simulink model "AN_Simulink_Model_v1"  (R2019b)
settings: Solver=VariableStepAuto  StartTime=0.0  StopTime=testtime  RelTol=1e-3
InitFcn:
  | AN_InitFcn_Callback
StopFcn:
  | AN_StopFcn_Callback
values from neighbouring files (symbols this model uses):
  alpha1 = 1.5e-6*100e3    (= 0.15)    [AN_Get_Model_Parameters.m]
  alpha2 = 1e-2*100e3    (= 1000)    [AN_Get_Model_Parameters.m]
  C1initphase = C1initphase + atan(CF/(-rzero))-atan((CF-pimag(2*i-1))/(-preal(2*i-1)))-atan((CF+pimag(2*i-1))/(-preal(2*i-1)))    [AN_Get_Model_Parameters.m]
  c1LPihc = ( Cihc - 2*pi*Fcihc ) / ( Cihc + 2*pi*Fcihc )    [AN_Get_Model_Parameters.m]
  c1LPohc = ( Cohc - 2*pi*Fcohc ) / ( Cohc + 2*pi*Fcohc )    [AN_Get_Model_Parameters.m]
  C1slope = 0.1    [AN_Get_Model_Parameters.m]
  c2LPihc = 2*pi*Fcihc / (2*pi*Fcihc + Cihc)    [AN_Get_Model_Parameters.m]
  c2LPohc = 2*pi*Fcohc / (2*pi*Fcohc + Cohc)    [AN_Get_Model_Parameters.m]
  C2slope = 0.2    [AN_Get_Model_Parameters.m]
  centerfreq = 165.4*(10^((bmplace+1.2)/(35/2.1)) - 1.0)    [AN_Get_Model_Parameters.m]
  CF = 2*pi*cf    [AN_Get_Model_Parameters.m]
  cf_factor = min(cfsat, 10^(cfslope*cf/1e3 + cfconst)) * 2.0    [AN_Get_Model_Parameters.m]
  cordiciterationswb = 52    [AN_Get_Model_Parameters.m]
  delta_phase = -2*pi*centerfreq*tdres    [AN_Get_Model_Parameters.m]
  fs_bilinear = 2*pi*cf/tan(2*pi*cf*tdres/2)    [AN_Get_Model_Parameters.m]
  gainihc = 1.0    (= 1)    [AN_Get_Model_Parameters.m]
  gainohc = 1.0    (= 1)    [AN_Get_Model_Parameters.m]
  ihcasym = 3.0    (= 3)    [AN_Get_Model_Parameters.m]
  m11 = 1/(C^2+5.9761e+003*C+2.5255e+007)    [AN_Get_Model_Parameters.m]
  m12 = -2*C^2+2*2.5255e+007    [AN_Get_Model_Parameters.m]
  m13 = C^2-5.9761e+003*C+2.5255e+007    [AN_Get_Model_Parameters.m]
  m14 = C^2+5.6665e+003*C    [AN_Get_Model_Parameters.m]
  m15 = -2*C^2    [AN_Get_Model_Parameters.m]
  m16 = C^2-5.6665e+003*C    [AN_Get_Model_Parameters.m]
  m21 = 1/(C^2+6.4255e+003*C+1.3975e+008)    [AN_Get_Model_Parameters.m]
  m22 = -2*C^2+2*1.3975e+008    [AN_Get_Model_Parameters.m]
  m23 = C^2-6.4255e+003*C+1.3975e+008    [AN_Get_Model_Parameters.m]
  m24 = C^2+5.8934e+003*C+1.7926e+008    [AN_Get_Model_Parameters.m]
  m25 = -2*C^2+2*1.7926e+008    [AN_Get_Model_Parameters.m]
  m26 = C^2-5.8934e+003*C+1.7926e+008    [AN_Get_Model_Parameters.m]
  m31 = 1/(C^2+2.4891e+004*C+1.2700e+009)    [AN_Get_Model_Parameters.m]
  m32 = -2*C^2+2*1.2700e+009    [AN_Get_Model_Parameters.m]
  m33 = C^2-2.4891e+004*C+1.2700e+009    [AN_Get_Model_Parameters.m]
  m34 = (3.1137e+003*C+6.9768e+008)    [AN_Get_Model_Parameters.m]
  m35 = 2*6.9768e+008    (= 1395360000)    [AN_Get_Model_Parameters.m]
  m36 = -3.1137e+003*C+6.9768e+008    [AN_Get_Model_Parameters.m]
  megainmax = 2    [AN_Get_Model_Parameters.m]
  minR = 0.05    [AN_Get_Model_Parameters.m]
  multFac = max(2.95*max(1.0,1.5-spont/100), 4.3-0.2*cf/1e3)    [AN_Get_Model_Parameters.m]
  norm_gainc1 = single(norm_gainc1)    [AN_Get_Model_Parameters.m]
  nSites = single(4)    [AN_Get_Model_Parameters.m]
  ohcasym = 7.0    (= 7)    [AN_Get_Model_Parameters.m]
  order_of_zero = half_order_pole    (= 5)    [AN_Get_Model_Parameters.m]
  pimag = zeros(11,1)    [AN_Get_Model_Parameters.m]
  preal = zeros(11,1)    [AN_Get_Model_Parameters.m]
  s0 = 12.0    (= 12)    [AN_Get_Model_Parameters.m]
  s1 = 5.0    (= 5)    [AN_Get_Model_Parameters.m]
  shift = 1.0/(1.0+ohcasym)    (= 0.125)    [AN_Get_Model_Parameters.m]
  spont = 100    [AN_Get_Model_Parameters.m]
  strength = (20.0e6)/(10^(corner/20))    (= 2000)    [AN_Get_Model_Parameters.m]
  tauwb = TauWBMax + (bmTaubm-bmTaumax)*(TauWBMax-TauWBMin)/(bmTaumax-bmTaumin)    [AN_Get_Model_Parameters.m]
  TauWBMax = Taumin + 0.2*(Taumax-Taumin)    [AN_Get_Model_Parameters.m]
  TauWBMin = TauWBMax/Taumax*Taumin    [AN_Get_Model_Parameters.m]
  wborder = 3    [AN_Get_Model_Parameters.m]
  x0 = s0*log((1.0/shift-1)/(1+exp(x1/s1)))    [AN_Get_Model_Parameters.m]
  x1 = 5.0    (= 5)    [AN_Get_Model_Parameters.m]
undefined symbols (not defined in the file or in its folder): bmTaumax, bmTaumin, cf, cihc, cohc, dfilt, Fs, jsin, norm_gainc2, tabs, tdres, trel, wbgain
libraries: dsparch4 x7, simulink x6, dspsrcs4 x3
(part 2 of 2)

== system AN_Simulink_Model_v1/Auditory Nerve Model/Subsystem/IHC LP Filter ==
  stimulus : Inport  OutDataTypeStr=single
  Biquad Filter1 : dsparch4/Biquad Filter  FilterSource=Dialog parameters  CoeffSource=Specify via dialog  FilterObject=dfilt.df2tsos([1 0.3 0.4],[1 0.1 0.2])  IIRFiltStruct=Direct form II transposed  BiQuadCoeffs=[c2LPihc c2LPihc 0 1 -c1LPihc 0; c2LPihc c2LPihc 0 1 -c1LPihc 0; c2LPihc c2LPihc 0 1 -c1LPihc 0]  ScaleValues=1  IC=0  ICnum=0  ICden=0  a0Flag=Warning  optimizeScaleValues=on  ScaleValueMode=Specify via input port (g)  roundingMode=Floor  overflowMode=on  scaleValueFracLength=14  denProdOutputFracLength=30  denAccumFracLength=30  secondMemoryFracLength=15
      settings: SourceProductName=DSP System Toolbox
  Biquad Filter4 : dsparch4/Biquad Filter  FilterSource=Dialog parameters  CoeffSource=Specify via dialog  FilterObject=dfilt.df2tsos([1 0.3 0.4],[1 0.1 0.2])  IIRFiltStruct=Direct form II transposed  BiQuadCoeffs=[gainihc*c2LPihc gainihc*c2LPihc 0 1 -c1LPihc 0; c2LPihc c2LPihc 0 1 -c1LPihc 0; c2LPihc c2LPihc 0 1 -c1LPihc 0;c2LPihc c2LPihc 0 1 -c1LPihc 0]  ScaleValues=1  IC=0  ICnum=0  ICden=0  a0Flag=Warning  optimizeScaleValues=on  ScaleValueMode=Specify via input port (g)  roundingMode=Floor  overflowMode=on  scaleValueFracLength=14  denProdOutputFracLength=30  denAccumFracLength=30  secondMemoryFracLength=15
      settings: SourceProductName=DSP System Toolbox
  output : Outport  VectorParamsAs1DForOutWhenUnconnected=off
  wires:
  stimulus/1 -> Biquad Filter4/1
  Biquad Filter4/1 -> Biquad Filter1/1  "output"
  Biquad Filter1/1 -> output/1  "output"

== system AN_Simulink_Model_v1/Auditory Nerve Model/Subsystem1/Calculate tauc1 ==
  note: Calculate final Time Constant which will be fed forward into C1 filter
  In1 : Inport
  Add : Sum
  Constant : Constant  Value=cohc  OutDataTypeStr=single  SampleTime=-1
  Constant1 : Constant  Value=bmTaumin  OutDataTypeStr=single  SampleTime=-1
  Constant2 : Constant  Value=bmTaumin  OutDataTypeStr=single  SampleTime=-1
  Product : Product
  Subtract : Sum  Inputs=+-
  Out1 : Outport  VectorParamsAs1DForOutWhenUnconnected=off
  wires:
  In1/1 -> Subtract/1  "tmptauc1"
  Constant/1 -> Product/1
  Constant1/1 -> Subtract/2
  Product/1 -> Add/1
  Add/1 -> Out1/1  "tauc1"
  Subtract/1 -> Product/2
  Constant2/1 -> Add/2

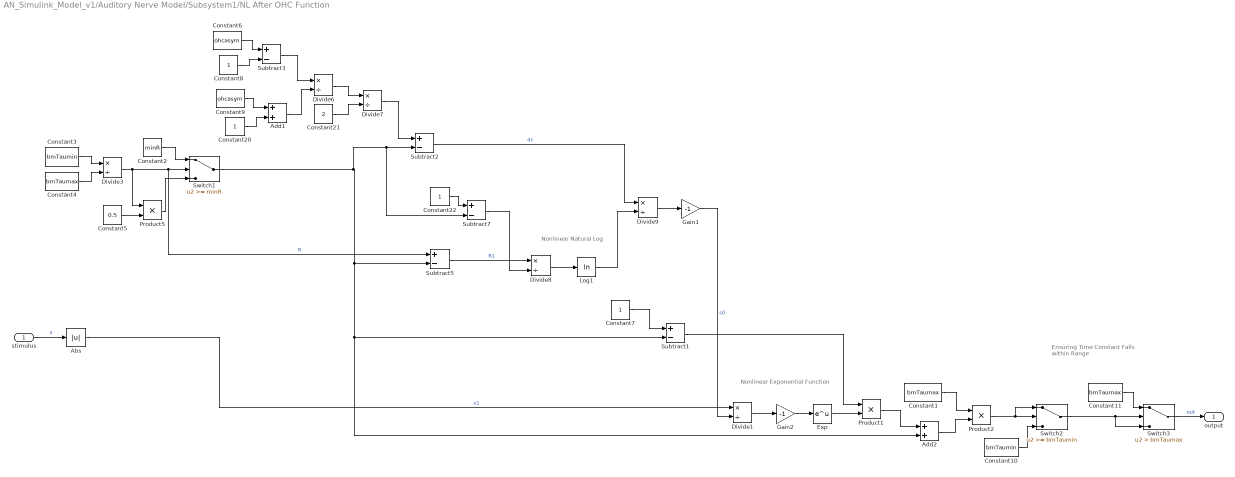
== system AN_Simulink_Model_v1/Auditory Nerve Model/Subsystem1/NL After OHC Function ==
  note: Ensuring Time Constant Falls within Range
  note: Nonlinear Natural Log
  note: Nonlinear Exponential Function
  stimulus : Inport
  Abs : Abs
  Add1 : Sum
  Add2 : Sum
  Constant1 : Constant  Value=bmTaumax  OutDataTypeStr=single  SampleTime=-1
  Constant10 : Constant  Value=bmTaumin  OutDataTypeStr=single  SampleTime=-1
  Constant11 : Constant  Value=bmTaumax  OutDataTypeStr=single  SampleTime=-1
  Constant2 : Constant  Value=minR  OutDataTypeStr=single  SampleTime=-1
  Constant{7..8,20,22} (4 alike) : Constant  OutDataTypeStr=single  SampleTime=-1
  Constant21 : Constant  Value=2  OutDataTypeStr=single  SampleTime=-1
  Constant3 : Constant  Value=bmTaumin  OutDataTypeStr=single  SampleTime=-1
  Constant4 : Constant  Value=bmTaumax  OutDataTypeStr=single  SampleTime=-1
  Constant5 : Constant  Value=0.5  OutDataTypeStr=single  SampleTime=-1
  Constant6 : Constant  Value=ohcasym  OutDataTypeStr=single  SampleTime=-1
  Constant9 : Constant  Value=ohcasym  OutDataTypeStr=single  SampleTime=-1
  Divide{1,3,6..9} (6 alike) : Product  Inputs=*/  SaturateOnIntegerOverflow=on  RndMeth=Zero
  Exp : Math  SaturateOnIntegerOverflow=on
  Gain1 : Gain  Gain=-1
  Gain2 : Gain  Gain=-1
  Log1 : Math  Operator=log  SaturateOnIntegerOverflow=on
  Product1 : Product
  Product2 : Product
  Product5 : Product
  Subtract{1..3,5,7} (5 alike) : Sum  Inputs=+-
  Switch1 : Switch  Threshold=minR
  Switch2 : Switch  Threshold=bmTaumin
  Switch3 : Switch  Criteria=u2 > Threshold  Threshold=bmTaumax
  output : Outport  VectorParamsAs1DForOutWhenUnconnected=off
  wires:
  Constant3/1 -> Divide3/1
  Constant4/1 -> Divide3/2
  Divide3/1 -> Subtract5/1, Switch1/2, Product5/1  "R"
  Constant2/1 -> Switch1/1
  Constant5/1 -> Product5/2
  Product5/1 -> Switch1/3
  Switch1/1 -> Subtract7/2, Subtract2/2, Add2/2, Subtract1/2, Subtract5/2
  Constant8/1 -> Subtract3/2
  Constant6/1 -> Subtract3/1
  Constant20/1 -> Add1/2
  Constant9/1 -> Add1/1
  Subtract3/1 -> Divide6/1
  Add1/1 -> Divide6/2
  Divide6/1 -> Divide7/1
  Constant21/1 -> Divide7/2
  Divide7/1 -> Subtract2/1
  Subtract2/1 -> Divide9/1  "dc"
  Subtract5/1 -> Divide8/1  "R1"
  Constant22/1 -> Subtract7/1
  Subtract7/1 -> Divide8/2
  Divide8/1 -> Log1/1
  Log1/1 -> Divide9/2
  Divide9/1 -> Gain1/1
  Gain1/1 -> Divide1/2  "s0"
  stimulus/1 -> Abs/1  "x"
  Abs/1 -> Divide1/1  "x1"
  Constant7/1 -> Subtract1/1
  Divide1/1 -> Gain2/1
  Gain2/1 -> Exp/1
  Subtract1/1 -> Product1/1
  Exp/1 -> Product1/2
  Product1/1 -> Add2/1
  Constant1/1 -> Product2/1
  Add2/1 -> Product2/2
  Product2/1 -> Switch2/1, Switch2/2
  Constant10/1 -> Switch2/3
  Switch2/1 -> Switch3/3, Switch3/2
  Constant11/1 -> Switch3/1
  Switch3/1 -> output/1  "out"

== system AN_Simulink_Model_v1/Auditory Nerve Model/Subsystem1/OHC LP Filter ==
  stimulus : Inport
  Biquad Filter4 : dsparch4/Biquad Filter  FilterSource=Dialog parameters  CoeffSource=Specify via dialog  FilterObject=dfilt.df2tsos([1 0.3 0.4],[1 0.1 0.2])  IIRFiltStruct=Direct form II transposed  BiQuadCoeffs=[gainohc*c2LPohc gainohc*c2LPohc 0 1 -c1LPohc 0; gainohc*c2LPohc gainohc*c2LPohc 0 1 -c1LPohc 0]  ScaleValues=1  IC=0  ICnum=0  ICden=0  a0Flag=Warning  optimizeScaleValues=on  ScaleValueMode=Specify via input port (g)  roundingMode=Floor  overflowMode=on  scaleValueFracLength=14  denProdOutputFracLength=30  denAccumFracLength=30  secondMemoryFracLength=15
      settings: SourceProductName=DSP System Toolbox
  output : Outport  VectorParamsAs1DForOutWhenUnconnected=off
  wires:
  stimulus/1 -> Biquad Filter4/1
  Biquad Filter4/1 -> output/1  "output"

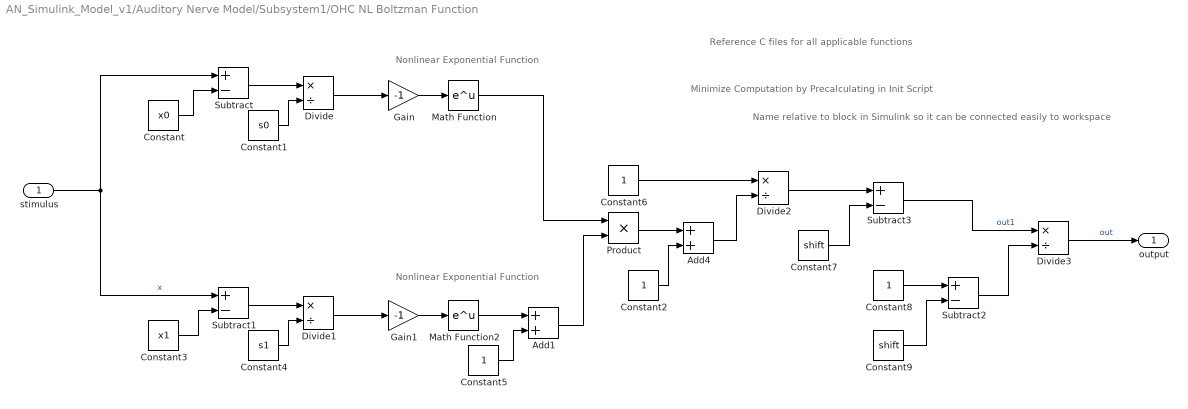
== system AN_Simulink_Model_v1/Auditory Nerve Model/Subsystem1/OHC NL Boltzman Function ==
  note: Name relative to block in Simulink so it can be connected easily to workspace
  note: Minimize Computation by Precalculating in Init Script
  note: Reference C files for all applicable functions
  note: Nonlinear Exponential Function
  note: Nonlinear Exponential Function
  stimulus : Inport
  Add1 : Sum
  Add4 : Sum
  Constant : Constant  Value=x0  OutDataTypeStr=single  SampleTime=-1
  Constant1 : Constant  Value=s0  OutDataTypeStr=single  SampleTime=-1
  Constant{2,5..6,8} (4 alike) : Constant  OutDataTypeStr=single  SampleTime=-1
  Constant3 : Constant  Value=x1  OutDataTypeStr=single  SampleTime=-1
  Constant4 : Constant  Value=s1  OutDataTypeStr=single  SampleTime=-1
  Constant7 : Constant  Value=shift  OutDataTypeStr=single  SampleTime=-1
  Constant9 : Constant  Value=shift  OutDataTypeStr=single  SampleTime=-1
  Divide{,1..3} (4 alike) : Product  Inputs=*/  SaturateOnIntegerOverflow=on  RndMeth=Zero
  Gain : Gain  Gain=-1
  Gain1 : Gain  Gain=-1
  Math Function : Math  SaturateOnIntegerOverflow=on
  Math Function2 : Math  SaturateOnIntegerOverflow=on
  Product : Product
  Subtract{,1..3} (4 alike) : Sum  Inputs=+-
  output : Outport  VectorParamsAs1DForOutWhenUnconnected=off
  wires:
  Constant/1 -> Subtract/2
  stimulus/1 -> Subtract1/1, Subtract/1  "x"
  Subtract/1 -> Divide/1
  Constant1/1 -> Divide/2
  Divide/1 -> Gain/1
  Gain/1 -> Math Function/1
  Constant3/1 -> Subtract1/2
  Subtract1/1 -> Divide1/1
  Constant4/1 -> Divide1/2
  Divide1/1 -> Gain1/1
  Gain1/1 -> Math Function2/1
  Math Function2/1 -> Add1/1
  Constant5/1 -> Add1/2
  Add1/1 -> Product/2
  Constant6/1 -> Divide2/1
  Divide2/1 -> Subtract3/1
  Constant7/1 -> Subtract3/2
  Subtract3/1 -> Divide3/1  "out1"
  Constant8/1 -> Subtract2/1
  Constant9/1 -> Subtract2/2
  Subtract2/1 -> Divide3/2
  Divide3/1 -> output/1  "out"
  Math Function/1 -> Product/1
  Product/1 -> Add4/1
  Constant2/1 -> Add4/2
  Add4/1 -> Divide2/2

== system AN_Simulink_Model_v1/Auditory Nerve Model/Synapse Model/NL Before PLA ==
  ihcout : Inport
  Abs : Abs
  Add2 : Sum
  Compare To Zero : simulink/Logic and Bit Operations/Compare To Zero  relop=>  OutDataTypeStr=boolean
  Constant6 : Constant  Value=0  OutDataTypeStr=single  SampleTime=-1
  Constant7 : Constant  Value=3*spont  OutDataTypeStr=single  SampleTime=-1
  Subsystem : Subsystem
  Switch : Switch  Criteria=u2 > Threshold  OutDataTypeStr=single
  powerLawIn : Outport  VectorParamsAs1DForOutWhenUnconnected=off
  wires:
  Constant6/1 -> Switch/3
  Switch/1 -> Add2/1
  Constant7/1 -> Add2/2
  Add2/1 -> powerLawIn/1
  ihcout/1 -> Subsystem/1(In1), Abs/1
  Subsystem/1(mappingOut) -> Switch/1
  Compare To Zero/1 -> Subsystem/Enable, Switch/2
  Abs/1 -> Compare To Zero/1, Subsystem/2(In2)

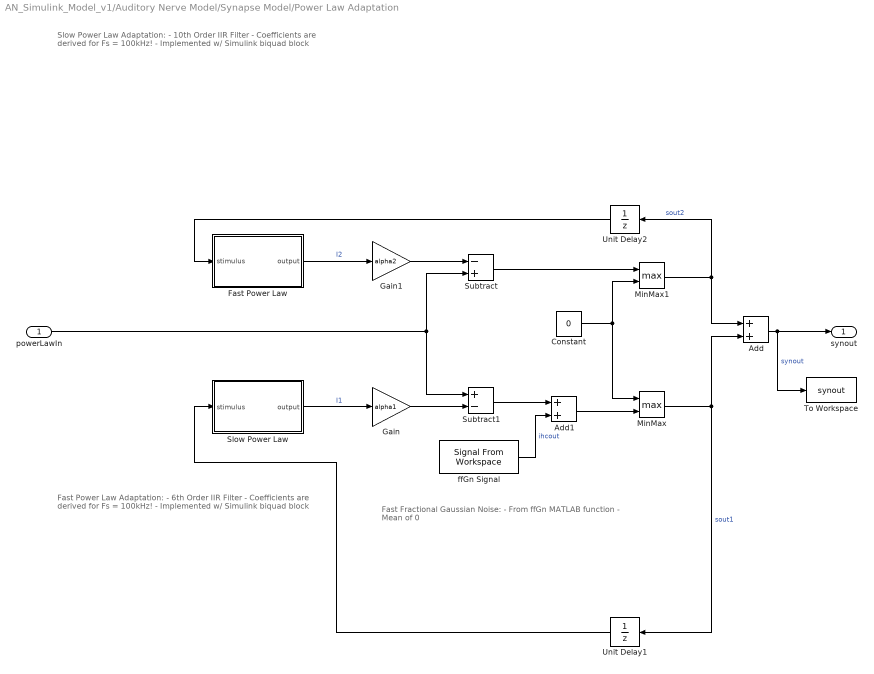
== system AN_Simulink_Model_v1/Auditory Nerve Model/Synapse Model/Power Law Adaptation ==
  note: Fast Power Law Adaptation:
      |
      | - 6th Order IIR Filter
      |
      | - Coefficients are derived for Fs = 100kHz!
      |
      | - Implemented w/ Simulink biquad block
  note: Slow Power Law Adaptation:
      |
      | - 10th Order IIR Filter
      |
      | - Coefficients are derived for Fs = 100kHz!
      |
      | - Implemented w/ Simulink biquad block
  note: Fast Fractional Gaussian Noise:
      |
      | - From ffGn MATLAB function
      |
      | - Mean of 0
  powerLawIn : Inport
  Add : Sum
  Add1 : Sum
  Constant : Constant  Value=0  OutDataTypeStr=single  SampleTime=-1
  Fast Power Law : Subsystem
  Gain : Gain  Gain=alpha1  ParamDataTypeStr=single  OutDataTypeStr=single
  Gain1 : Gain  Gain=alpha2  ParamDataTypeStr=single  OutDataTypeStr=single
  MinMax : MinMax  Function=max  Inputs=2
  MinMax1 : MinMax  Function=max  Inputs=2
  Slow Power Law : Subsystem
  Subtract : Sum  Inputs=-+
  Subtract1 : Sum  Inputs=+-
  To Workspace : ToWorkspace  VariableName=synout  SampleTime=-1
      settings: Save2DSignal=2-D array (concatenate along first dimension)
  Unit Delay1 : UnitDelay  SampleTime=-1  HasFrameUpgradeWarning=on
  Unit Delay2 : UnitDelay  SampleTime=-1  HasFrameUpgradeWarning=on
  ffGn Signal : dspsrcs4/Signal From Workspace  X=noise  Ts=1/Fs  nsamps=1  OutputAfterFinalValue=Setting to zero  ignoreOrWarnInputAndFrameLengths=off  OutputFrames=off
  synout : Outport  VectorParamsAs1DForOutWhenUnconnected=off
  wires:
  Gain/1 -> Subtract1/2
  Subtract/1 -> MinMax1/1
  MinMax1/1 -> Unit Delay2/1, Add/1  "sout2"
  Add/1 -> synout/1, To Workspace/1  "synout"
  powerLawIn/1 -> Subtract/2, Subtract1/1
  Fast Power Law/1(output) -> Gain1/1  "I2"
  Unit Delay2/1 -> Fast Power Law/1(stimulus)
  Slow Power Law/1(output) -> Gain/1  "I1"
  Subtract1/1 -> Add1/1
  Constant/1 -> MinMax/1, MinMax1/2
  MinMax/1 -> Unit Delay1/1, Add/2  "sout1"
  Unit Delay1/1 -> Slow Power Law/1(stimulus)
  Gain1/1 -> Subtract/1
  Add1/1 -> MinMax/2
  ffGn Signal/1 -> Add1/2  "ihcout"

== system AN_Simulink_Model_v1/Auditory Nerve Model/f(tauc1)/Calculate tauwb ==
  In1 : Inport
  Add : Sum
  Constant1 : Constant  Value=bmTaumax  OutDataTypeStr=single  SampleTime=-1
  Constant2 : Constant  Value=TauWBMax  OutDataTypeStr=single  SampleTime=-1
  Constant3 : Constant  Value=TauWBMax  OutDataTypeStr=single  SampleTime=-1
  Constant4 : Constant  Value=TauWBMin  OutDataTypeStr=single  SampleTime=-1
  Constant5 : Constant  Value=bmTaumax  OutDataTypeStr=single  SampleTime=-1
  Constant6 : Constant  Value=bmTaumin  OutDataTypeStr=single  SampleTime=-1
  Divide : Product  Inputs=*/  SaturateOnIntegerOverflow=on  RndMeth=Zero
  Product : Product
  Subtract : Sum  Inputs=+-
  Subtract1 : Sum  Inputs=+-
  Subtract2 : Sum  Inputs=+-
  Out1 : Outport  OutDataTypeStr=single  VectorParamsAs1DForOutWhenUnconnected=off
  wires:
  In1/1 -> Subtract/1  "tauc1"
  Constant1/1 -> Subtract/2
  Product/1 -> Add/1
  Subtract/1 -> Product/1
  Constant3/1 -> Subtract1/1
  Constant4/1 -> Subtract1/2
  Constant6/1 -> Subtract2/2
  Constant5/1 -> Subtract2/1
  Subtract2/1 -> Divide/2
  Subtract1/1 -> Divide/1
  Divide/1 -> Product/2
  Constant2/1 -> Add/2
  Add/1 -> Out1/1

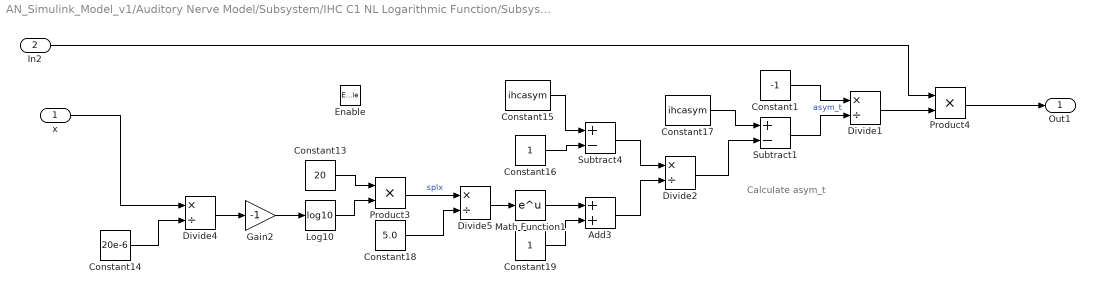
== system AN_Simulink_Model_v1/Auditory Nerve Model/Subsystem/IHC C1 NL Logarithmic Function/Subsystem ==
  note: Calculate asym_t
  x : Inport
  In2 : Inport  Port=2
  Enable : EnablePort
  Add3 : Sum
  Constant1 : Constant  Value=-1  OutDataTypeStr=single  SampleTime=-1
  Constant13 : Constant  Value=20  OutDataTypeStr=single  SampleTime=-1
  Constant14 : Constant  Value=20e-6  OutDataTypeStr=single  SampleTime=-1
  Constant15 : Constant  Value=ihcasym  OutDataTypeStr=single  SampleTime=-1
  Constant16 : Constant  OutDataTypeStr=single  SampleTime=-1
  Constant17 : Constant  Value=ihcasym  OutDataTypeStr=single  SampleTime=-1
  Constant18 : Constant  Value=5.0  OutDataTypeStr=single  SampleTime=-1
  Constant19 : Constant  OutDataTypeStr=single  SampleTime=-1
  Divide{1..2,4..5} (4 alike) : Product  Inputs=*/  SaturateOnIntegerOverflow=on  RndMeth=Zero
  Gain2 : Gain  Gain=-1
  Log10 : Math  Operator=log10  SaturateOnIntegerOverflow=on
  Math Function1 : Math  SaturateOnIntegerOverflow=on
  Product3 : Product
  Product4 : Product
  Subtract1 : Sum  Inputs=+-
  Subtract4 : Sum  Inputs=+-
  Out1 : Outport  OutDataTypeStr=single  SourceOfInitialOutputValue=Input signal  OutputWhenDisabled=reset
  wires:
  Gain2/1 -> Log10/1
  Constant13/1 -> Product3/1
  Divide5/1 -> Math Function1/1
  Math Function1/1 -> Add3/1
  Product3/1 -> Divide5/1  "splx"
  Constant15/1 -> Subtract4/1
  Log10/1 -> Product3/2
  Constant14/1 -> Divide4/2
  Constant19/1 -> Add3/2
  Divide4/1 -> Gain2/1
  Constant18/1 -> Divide5/2
  Subtract4/1 -> Divide2/1
  Constant17/1 -> Subtract1/1
  Add3/1 -> Divide2/2
  Divide2/1 -> Subtract1/2
  Subtract1/1 -> Divide1/2  "asym_t"
  Constant1/1 -> Divide1/1
  Constant16/1 -> Subtract4/2
  Divide1/1 -> Product4/2
  In2/1 -> Product4/1
  x/1 -> Divide4/1
  Product4/1 -> Out1/1

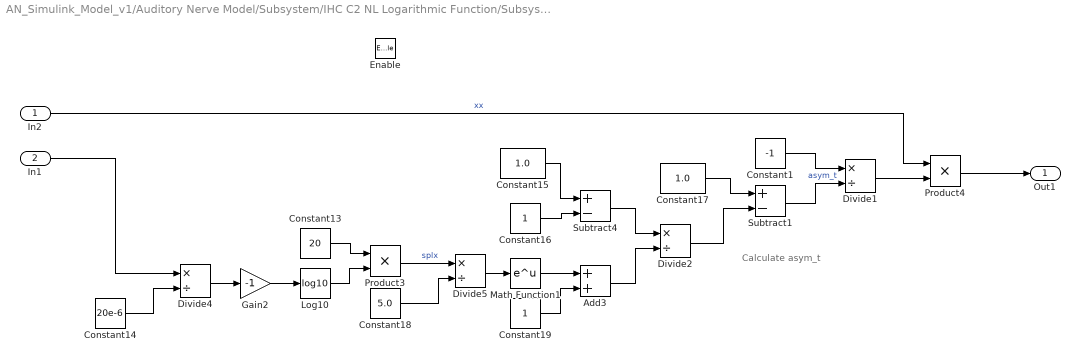
== system AN_Simulink_Model_v1/Auditory Nerve Model/Subsystem/IHC C2 NL Logarithmic Function/Subsystem ==
  note: Calculate asym_t
  In2 : Inport
  In1 : Inport  Port=2
  Enable : EnablePort
  Add3 : Sum
  Constant1 : Constant  Value=-1  OutDataTypeStr=single  SampleTime=-1
  Constant13 : Constant  Value=20  OutDataTypeStr=single  SampleTime=-1
  Constant14 : Constant  Value=20e-6  OutDataTypeStr=single  SampleTime=-1
  Constant15 : Constant  Value=1.0  OutDataTypeStr=single  SampleTime=-1
  Constant16 : Constant  OutDataTypeStr=single  SampleTime=-1
  Constant17 : Constant  Value=1.0  OutDataTypeStr=single  SampleTime=-1
  Constant18 : Constant  Value=5.0  OutDataTypeStr=single  SampleTime=-1
  Constant19 : Constant  OutDataTypeStr=single  SampleTime=-1
  Divide{1..2,4..5} (4 alike) : Product  Inputs=*/  SaturateOnIntegerOverflow=on  RndMeth=Zero
  Gain2 : Gain  Gain=-1
  Log10 : Math  Operator=log10  SaturateOnIntegerOverflow=on
  Math Function1 : Math  SaturateOnIntegerOverflow=on
  Product3 : Product
  Product4 : Product
  Subtract1 : Sum  Inputs=+-
  Subtract4 : Sum  Inputs=+-
  Out1 : Outport  SourceOfInitialOutputValue=Input signal  OutputWhenDisabled=reset
  wires:
  Constant18/1 -> Divide5/2
  Divide4/1 -> Gain2/1
  Divide1/1 -> Product4/2
  Constant13/1 -> Product3/1
  Constant14/1 -> Divide4/2
  Constant16/1 -> Subtract4/2
  Constant1/1 -> Divide1/1
  Add3/1 -> Divide2/2
  Constant17/1 -> Subtract1/1
  Constant19/1 -> Add3/2
  Constant15/1 -> Subtract4/1
  Product3/1 -> Divide5/1  "splx"
  Divide5/1 -> Math Function1/1
  Subtract4/1 -> Divide2/1
  Gain2/1 -> Log10/1
  Subtract1/1 -> Divide1/2  "asym_t"
  Log10/1 -> Product3/2
  Math Function1/1 -> Add3/1
  Divide2/1 -> Subtract1/2
  In2/1 -> Product4/1  "xx"
  Product4/1 -> Out1/1
  In1/1 -> Divide4/1

== system AN_Simulink_Model_v1/Auditory Nerve Model/Synapse Model/NL Before PLA/Subsystem ==
  note: Nonlinear log
  note: Nonlinear power
  In1 : Inport
  In2 : Inport  Port=2
  Enable : EnablePort
  Add : Sum
  Constant : Constant  Value=cf_factor  OutDataTypeStr=single  SampleTime=-1
  Constant1 : Constant  Value=multFac  OutDataTypeStr=single  SampleTime=-1
  Constant2 : Constant  OutDataTypeStr=single  SampleTime=-1
  Constant3 : Constant  Value=-1  OutDataTypeStr=single  SampleTime=-1
  Gain : Gain  Gain=0.9
  Log10 : Math  Operator=log10  RndMeth=Zero  SaturateOnIntegerOverflow=on
  Pow : Math  Operator=10^u  RndMeth=Zero  SaturateOnIntegerOverflow=on
  Product : Product
  Product1 : Product
  Switch : Switch
  mappingOut : Outport
  wires:
  Constant3/1 -> Switch/3
  Switch/1 -> Product1/2
  Pow/1 -> Product1/1
  In1/1 -> Switch/2
  Constant/1 -> Product/2
  Product/1 -> Log10/1
  Constant2/1 -> Switch/1
  Log10/1 -> Gain/1
  Gain/1 -> Add/1
  Add/1 -> Pow/1
  Constant1/1 -> Add/2
  In2/1 -> Product/1
  Product1/1 -> mappingOut/1  "mappingOut"

== system AN_Simulink_Model_v1/Auditory Nerve Model/Synapse Model/Power Law Adaptation/Fast Power Law ==
  stimulus : Inport
  Biquad Filter1 : dsparch4/Biquad Filter  FilterSource=Dialog parameters  CoeffSource=Specify via dialog  FilterObject=dfilt.df2tsos([1 0.3 0.4],[1 0.1 0.2])  IIRFiltStruct=Direct form II transposed  BiQuadCoeffs=fast_coeffs  ScaleValues=1  IC=0  ICnum=0  ICden=0  a0Flag=Warning  optimizeScaleValues=on  ScaleValueMode=Specify via input port (g)  roundingMode=Floor  overflowMode=on  scaleValueFracLength=14  denProdOutputFracLength=30  denAccumFracLength=30  secondMemoryFracLength=15
      settings: SourceProductName=DSP System Toolbox
  output : Outport  VectorParamsAs1DForOutWhenUnconnected=off
  wires:
  stimulus/1 -> Biquad Filter1/1
  Biquad Filter1/1 -> output/1

== system AN_Simulink_Model_v1/Auditory Nerve Model/Synapse Model/Power Law Adaptation/Slow Power Law ==
  stimulus : Inport
  Biquad Filter1 : dsparch4/Biquad Filter  FilterSource=Dialog parameters  CoeffSource=Specify via dialog  FilterObject=dfilt.df2tsos([1 0.3 0.4],[1 0.1 0.2])  IIRFiltStruct=Direct form II transposed  BiQuadCoeffs=slow_coeffs  ScaleValues=1  IC=0  ICnum=0  ICden=0  a0Flag=Warning  optimizeScaleValues=on  ScaleValueMode=Specify via input port (g)  roundingMode=Floor  overflowMode=on  scaleValueFracLength=14  denProdOutputFracLength=30  denAccumFracLength=30  secondMemoryFracLength=15
      settings: SourceProductName=DSP System Toolbox
  output : Outport  VectorParamsAs1DForOutWhenUnconnected=off
  wires:
  stimulus/1 -> Biquad Filter1/1
  Biquad Filter1/1 -> output/1

== matlab function AN_Simulink_Model_v1/Auditory Nerve Model/f(tauc1)/gain_groupdelay ==
  data: tdres input; wb_gain output; centerfreq input; cf input; tau input; grdelay output
% gain_groupdelay() - A MATLAB function created to recreate the
% gain_groupdelay function implemented in the AN model C source code
%
% [wb_gain, grdelay] = gain_groupdelay(tdres, centerfreq, cf, tau)
%
% The function takes in the binsize, neuron shifted centerfrequency,
% neuron characteristic frequency, and time constant and returns the
% wideband gain and group delay of the control path

% Inputs:
%   tdres = binsize, or sampling period
%   centerfreq = neuron shifted center frequency according to basilar membrane location
%   cf = neuron characteristic frequency
%   tau = time constant parameter
%
% Outputs:
%   wb_gain = wideband filter control path gain
%   grdelay = control path group delay

% ---------------------------------------------------------------------- %

% Copyright 2019 Flat Earth Inc
%
% THE SOFTWARE IS PROVIDED "AS IS", WITHOUT WARRANTY OF ANY KIND, EXPRESS OR IMPLIED,
% INCLUDING BUT NOT LIMITED TO THE WARRANTIES OF MERCHANTABILITY, FITNESS FOR A PARTICULAR
% PURPOSE AND NONINFRINGEMENT. IN NO EVENT SHALL THE AUTHORS OR COPYRIGHT HOLDERS BE LIABLE
% FOR ANY CLAIM, DAMAGES OR OTHER LIABILITY, WHETHER IN AN ACTION OF CONTRACT, TORT OR OTHERWISE,
% ARISING FROM, OUT OF OR IN CONNECTION WITH THE SOFTWARE OR THE USE OR OTHER DEALINGS IN THE SOFTWARE.
%
% Matthew Blunt
% Flat Earth Inc
% 985 Technology Blvd
% Bozeman, MT 59718
% support@flatearthinc.com

% Auditory Nerve Simulink Model Code
% gain_groupdelay MATLAB Function
% 06/27/2019

% ---------------------------------------------------------------------- %

% Function copied from AN model C source code, with a few minor adjustments
% in order for the function to operate in MATLAB

function [wb_gain, grdelay] = gain_groupdelay(tdres, centerfreq, cf, tau)

  tmpcos = cos(2*pi*(centerfreq-cf)*tdres);
  dtmp2 = tau*2.0/tdres;
  c1LP = (dtmp2-1)/(dtmp2+1);
  c2LP = 1.0/(dtmp2+1);
  tmp1 = 1+c1LP*c1LP-2*c1LP*tmpcos;
  tmp2 = 2*c2LP*c2LP*(1+tmpcos);
  
  wb_gain = (tmp1/tmp2)^0.5;
  
  grdelay = floor((0.5-(c1LP^2-c1LP*tmpcos)/(1+c1LP^2-2*c1LP*tmpcos)));

end

== matlab function AN_Simulink_Model_v1/Auditory Nerve Model/CP Wideband Gammatone Filter/MATLAB Function1 ==
  data: phase input; wbphase output; delta_phase input
% Matthew Blunt
% Speech % Hearing Internship
% Check Gammatone Cosine Argument
% 6/6/2019

% ---------------------------------------------------------------------- %
% NOTES: 
% ---------------------------------------------------------------------- %

% The following script is designed to work within the CP Wideband Gammatone
% Filter Simulink model in order to ensure that the argument of the
% trigonometric representation of a complex exponential remains within
% [-2pi,2pi). The function will simply take in the wb phase variable and
% output the same value in radians that falls within the range of arguments
% for the Simulink trigonometric block.

% *** NOTE: Edited by Matthew Blunt 03/05/2020
% *** Now evaluates bounds in the feedback loop to ensure stability for
% FPGA implementation

% ---------------------------------------------------------------------- %
% CODE: 
% ---------------------------------------------------------------------- %

% *** Edited by Matthew Blunt 03/05/2020
% *** Only accounts for negative values of delta_phase
function wbphase = WbGammaToneCosineArgCheck(phase,delta_phase)
    if phase <= (-2*pi - delta_phase)
        phase = phase+2*pi;
    end
    wbphase = phase;
end

== stateflow chart AN_Simulink_Model_v1/Auditory Nerve Model/Spike Generator/Stateflow Logic Chart ==
  settings: updateMethod=DISCRETE  sampleTime=tdres  executeAtInitialization=1
  note: 1st Synaptic Site State
      |
      | - Updates according to whether the synaptic site is sensing input or is going through the redocking period.
  note: 2nd Synaptic Site State
      |
      | - Updates according to whether the synaptic site is sensing input or is going through the redocking period.
  note: 3rd Synaptic Site State
      |
      | - Updates according to whether the synaptic site is sensing input or is going through the redocking period.
  note: 4th Synaptic Site State
      |
      | - Updates according to whether the synaptic site is sensing input or is going through the redocking period.
  note: Redocking Decay State
      |
      | - Updates according to whether the redocking period should be decayed or a redocking event has occured during the time step
  note: Synaptic State
      |
      | - Updates according to whether the synapse is ready to fire or is going through the refractory period.
  state SynapticSite1 [parallel]
    settings: executionOrder=2
    note: Synaptic Site Sensing Input
    note: Synaptic Site In Redocking Period
    note: Default Transition
    state SenseInput
      entry:
      redockStatus1 = single(0);
      Xsum1 = Xsum1 + synout/(single(4));
      releaseStatus1 = checkRelease(Xsum1, unitRateInterval1);
      during:
      Xsum1 = Xsum1 + synout/(single(4));
      releaseStatus1 = checkRelease(Xsum1, unitRateInterval1);
      exit:
      oneSiteRedock1 = getNewRedock(current_redocking_period, randNums);
      Xsum1= single(0);
      unitRateInterval1 = getNewUnitRateInterval(randNums);
    state RedockPeriod
      entry:
      elapsed_time1 = single(0);
      redockStatus1 = checkRedock(elapsed_time1, oneSiteRedock1);
      elapsed_time1  = elapsed_time1 + tdres;
      releaseStatus1 = single(0);
      during:
      redockStatus1 = checkRedock(elapsed_time1, oneSiteRedock1);
      elapsed_time1 = elapsed_time1 + tdres;
      exit:
      elapsed_time1 = single(0);
      current_redocking_period = previous_redocking_period + t_rd_jump;
      previous_redocking_period = current_redocking_period;
    (default) -> SynapticSite1.RedockPeriod
    SynapticSite1.SenseInput -> SynapticSite1.RedockPeriod : [releaseStatus1 == single(1)]
    SynapticSite1.RedockPeriod -> SynapticSite1.SenseInput : [redockStatus1 == single(1)]
  state SynapticSite2 [parallel]
    settings: executionOrder=3
    note: Synaptic Site Sensing Input
    note: Synaptic Site In Redocking Period
    note: Default Transition
    state SenseInput
      entry:
      redockStatus2 = single(0);
      Xsum2 = Xsum2 + synout/(single(4));
      releaseStatus2 = checkRelease(Xsum2, unitRateInterval2);
      during:
      Xsum2 = Xsum2 + synout/(single(4));
      releaseStatus2 = checkRelease(Xsum2, unitRateInterval2);
      exit:
      oneSiteRedock2 = getNewRedock(current_redocking_period, randNums);
      Xsum2= single(0);
      unitRateInterval2 = getNewUnitRateInterval(randNums);
    state RedockPeriod
      entry:
      elapsed_time2 = single(0);
      redockStatus2 = checkRedock(elapsed_time2, oneSiteRedock2);
      elapsed_time2  = elapsed_time2 + tdres;
      releaseStatus2 = single(0);
      during:
      redockStatus2 = checkRedock(elapsed_time2, oneSiteRedock2);
      elapsed_time2 = elapsed_time2 + tdres;
      exit:
      elapsed_time2 = single(0);
      current_redocking_period = previous_redocking_period + t_rd_jump;
      previous_redocking_period = current_redocking_period;
    (default) -> SynapticSite2.RedockPeriod
    SynapticSite2.SenseInput -> SynapticSite2.RedockPeriod : [releaseStatus2 == single(1)]
    SynapticSite2.RedockPeriod -> SynapticSite2.SenseInput : [redockStatus2 == single(1)]
  state SynapticSite3 [parallel]
    settings: executionOrder=4
    note: Synaptic Site Sensing Input
    note: Synaptic Site In Redocking Period
    note: Default Transition
    state SenseInput
      entry:
      redockStatus3 = single(0);
      Xsum3 = Xsum3 + synout/(single(4));
      releaseStatus3 = checkRelease(Xsum3, unitRateInterval3);
      during:
      Xsum3 = Xsum3 + synout/(single(4));
      releaseStatus3 = checkRelease(Xsum3, unitRateInterval3);
      exit:
      oneSiteRedock3 = getNewRedock(current_redocking_period, randNums);
      Xsum3= single(0);
      unitRateInterval3 = getNewUnitRateInterval(randNums);
    state RedockPeriod
      entry:
      elapsed_time3 = single(0);
      redockStatus3 = checkRedock(elapsed_time3, oneSiteRedock3);
      elapsed_time3  = elapsed_time3 + tdres;
      releaseStatus3 = single(0);
      during:
      redockStatus3 = checkRedock(elapsed_time3, oneSiteRedock3);
      elapsed_time3 = elapsed_time3 + tdres;
      exit:
      elapsed_time3 = single(0);
      current_redocking_period = previous_redocking_period + t_rd_jump;
      previous_redocking_period = current_redocking_period;
    (default) -> SynapticSite3.RedockPeriod
    SynapticSite3.SenseInput -> SynapticSite3.RedockPeriod : [releaseStatus3 == single(1)]
    SynapticSite3.RedockPeriod -> SynapticSite3.SenseInput : [redockStatus3 == single(1)]
  state SynapticSite4 [parallel]
    settings: executionOrder=5
    note: Synaptic Site Sensing Input
    note: Synaptic Site In Redocking Period
    note: Default Transition
    state SenseInput
      entry:
      redockStatus4 = single(0);
      Xsum4 = Xsum4 + synout/(single(4));
      releaseStatus4 = checkRelease(Xsum4, unitRateInterval4);
      during:
      Xsum4 = Xsum4 + synout/(single(4));
      releaseStatus4 = checkRelease(Xsum4, unitRateInterval4);
      exit:
      oneSiteRedock4 = getNewRedock(current_redocking_period, randNums);
      Xsum4= single(0);
      unitRateInterval4 = getNewUnitRateInterval(randNums);
    state RedockPeriod
      entry:
      elapsed_time4 = single(0);
      redockStatus4 = checkRedock(elapsed_time4, oneSiteRedock4);
      elapsed_time4  = elapsed_time4 + tdres;
      releaseStatus4 = single(0);
      during:
      redockStatus4 = checkRedock(elapsed_time4, oneSiteRedock4);
      elapsed_time4 = elapsed_time4 + tdres;
      exit:
      elapsed_time4 = single(0);
      current_redocking_period = previous_redocking_period + t_rd_jump;
      previous_redocking_period = current_redocking_period;
    (default) -> SynapticSite4.RedockPeriod
    SynapticSite4.SenseInput -> SynapticSite4.RedockPeriod : [releaseStatus4 == single(1)]
    SynapticSite4.RedockPeriod -> SynapticSite4.SenseInput : [redockStatus4 == single(1)]
  state RedockingDecay [parallel]
    settings: executionOrder=6
    note: Decay Redocking Period
    note: Don't Decay Redocking Period
    note: Default Transition
    state DecayRedockingPeriod
      entry:
      current_redocking_period = decayRedock(previous_redocking_period, tdres, tau, t_rd_rest);
      previous_redocking_period = current_redocking_period;
      trd_vector = current_redocking_period;
      during:
      current_redocking_period = decayRedock(previous_redocking_period, tdres, tau, t_rd_rest);
      previous_redocking_period = current_redocking_period;
      trd_vector = current_redocking_period;
    state NoDecay
      entry:
      trd_vector = current_redocking_period;
      during:
      trd_vector = current_redocking_period;
    (default) -> DecayRedockingPeriod
    DecayRedockingPeriod -> NoDecay : [redockStatus1 == single(1) || redockStatus2 == single(1) || redockStatus3 == single(1) || redockStatus4 == single(1)]
    NoDecay -> DecayRedockingPeriod : [redockStatus1 == single(0) && redockStatus2 == single(0) && redockStatus3 == single(0) && redockStatus4 == single(0)]
  state Synapse [parallel]
    settings: executionOrder=1
    note: Synapse Ready to Fire
    note: Synapse in Refractory Period
    note: Default Transition
    state RefractoryPeriod
      entry:
      refractoryStatus = checkRefractory(refractory_time, Tref);
      refractory_time = refractory_time + tdres;
      during:
      sptime = single(0);
      refractoryStatus = checkRefractory(refractory_time, Tref);
      refractory_time = refractory_time + tdres;
      exit:
      refractory_time = single(0);
      sptime = single(0);
    state SynapseReady
      during:
      sptime = single(0);
      exit:
      sptime = single(1);
      spCount = spCount + single(1);
      Tref = getTref(synout, randNums, trel, tabs);
    (default) -> SynapseReady
    SynapseReady -> RefractoryPeriod : [releaseStatus1 == single(1) || releaseStatus2 == single(1) || releaseStatus3 == single(1) || releaseStatus4 == single(1)]
    RefractoryPeriod -> SynapseReady : [refractoryStatus == single(0)]
  note: Release Status Graphical Function
      |
      | Input : Sensing Input Sum (Xsum) & Release Threshold (unitRateInterval)
      |
      | Output : Release Status Condition (releaseStatus)
      |
      | - Checks if a Release Event Occurs for the Synaptic Site (1) or not (0)
  state releaseStatuscond = checkRelease(Xsumval, unitRateIntervalval) [function]
    (default) -> (junction 138) : % Check to see if a release event occurs.
    (junction 138) -> (junction 139) [order 1] : [Xsumval >= unitRateIntervalval]
    (junction 138) -> (junction 140) [order 2] : {releaseStatuscond = single(0);}
    (junction 139) -> (junction 141) : {releaseStatuscond = single(1);}
    (junction 141) -> (junction 140)
    (junction 140) -> (junction 142)
  state redockStatuscond = checkRedock(elapsed_timeval, oneSiteRedockval) [function]
    (default) -> (junction 153) : % Check to see if a redocking event occurs.
    (junction 153) -> (junction 154) [order 1] : [elapsed_timeval >= oneSiteRedockval]
    (junction 153) -> (junction 155) [order 2] : {redockStatuscond = single(0);}
    (junction 154) -> (junction 156) : {redockStatuscond = single(1);}
    (junction 156) -> (junction 155)
    (junction 155) -> (junction 157)
  note: Redock Status Graphical Function
      |
      | Input : Elapsed Time during Redocking Event (elapsed_time) & Site Specific Redocking Period (oneSiteRedock)
      |
      | Output : Redock Status Condition (redockStatus)
      |
      | - Checks if a Redocking Event Occurs for the Synaptic Site (1) or not (0)
  state refractoryStatuscond = checkRefractory(refractory_timeval, Trefval) [function]
    (default) -> (junction 272) : % Check to see if the synapse is in the refractory period.
    (junction 272) -> (junction 273) [order 1] : [refractory_timeval >= Trefval]
    (junction 272) -> (junction 274) [order 2] : {refractoryStatuscond = single(1);}
    (junction 273) -> (junction 275) : {refractoryStatuscond = single(0);}
    (junction 275) -> (junction 274)
    (junction 274) -> (junction 276)
  note: Refractory Status Graphical Function
      |
      | Input : Elapsed Time during Refractory Period (refractory_time) & Refractory Period (Tref)
      |
      | Output : Refractory Status Condition (refractoryStatus)
      |
      | - Checks if the Synapse is in the Refractory Period (1) or not (0)
  note: Get New Unit Rate Interval MATLAB Function
      |
      | Input : Uniformly Distributed Random Number between 0 and 1 (randNums)
      |
      | Output : New Release Threshold Value (unitRateInterval)
      |
      | - Calculates the New Release Threshold Value for the Synaptic Site after a Release Event
  note: Get New Site Specific Redocking Period MATLAB Function
      |
      | Input : Current Redocking Period (current_redocking_period) & Uniformly Distributed Random Number between 0 and 1 (randNums)
      |
      | Output : New Redocking Period for Specific Synaptic Site (oneSiteRedock)
      |
      | - Calculates the New Redocking Period for Specific Synaptic Site
  note: Decay Redocking Period MATLAB Function
      |
      | Input : Previous Redocking Period (previous_redocking_period), Sample Time (tdres),
      | Decay Time Constant (tau), & Resting Redocking Time (t_rd_rest)
      |
      | Output : Current Redocking Period (current_redocking_period)
      |
      | - Decays the Redocking Period for the Next TIme Step
  note: Get New Refractory Period MATLAB Function
      |
      | Input : Synapse Output (synout), Uniformly Distributed Random Number between 0 and 1 (randNums),
      | Relative Refractory Time (trel), & Absolute Refractory Time (tabs)
      |
      | Output : New Refractory Period for the Synapse (Tref)
      |
      | - Calculates the New Refractory Period for the Synapse
  data: Xsumval function_input single; releaseStatuscond function_output single; unitRateIntervalval function_input single; elapsed_timeval function_input single; redockStatuscond function_output single; oneSiteRedockval function_input single; refractory_timeval function_input single; refractoryStatuscond function_output single; Trefval function_input single; randNumsval function_input single; unitRateIntervalval function_output single; current_redocking_periodval function_input single; randNumsval function_input single; oneSiteRedockval function_output single; previous_redocking_periodval function_input single; current_redocking_periodval function_output single; tdresval function_input single; tauval function_input single; t_rd_restval function_input single; synoutval function_input single; Trefval function_output single; randNumsval function_input single; trelval function_input single; tabsval function_input single; tdres parameter single; synout input single; refractoryStatus local single; randNums input single; sptime output single; spCount output single; current_redocking_period output single; trd_vector output single; t_rd_jump parameter single; releaseStatus1 local single; redockStatus1 local single; releaseStatus4 local single; redockStatus4 local single; releaseStatus2 local single; redockStatus2 local single; releaseStatus3 local single; redockStatus3 local single; t_rd_rest parameter single; tau parameter single; trel parameter single; tabs parameter single; unitRateInterval4 local single; unitRateInterval3 local single; unitRateInterval2 local single; unitRateInterval1 local single; oneSiteRedock4 local single; oneSiteRedock3 local single; oneSiteRedock2 local single; oneSiteRedock1 local single; elapsed_time4 local single; elapsed_time3 local single; elapsed_time2 local single; elapsed_time1 local single; Xsum4 local single; Xsum3 local single; Xsum2 local single; Xsum1 local single; Tref local single; previous_redocking_period local single; refractory_time local single
  function unitRateIntervalval = getNewUnitRateInterval(randNumsval):
    | function unitRateIntervalval = getNewUnitRateInterval(randNumsval)
    |     unitRateIntervalval = single(-log(randNumsval)/tdres);
    | end
  function oneSiteRedockval = getNewRedock(current_redocking_periodval, randNumsval):
    | function oneSiteRedockval = getNewRedock(current_redocking_periodval, randNumsval)
    |     oneSiteRedockval = single(-current_redocking_periodval * log(randNumsval));
    | end
  function current_redocking_periodval = decayRedock(previous_redocking_periodval,tdresval,tauval,t_rd_restval):
    | function current_redocking_periodval = decayRedock(previous_redocking_periodval,tdresval,tauval,t_rd_restval)
    |     current_redocking_periodval = single(previous_redocking_periodval - (tdresval/tauval)*(previous_redocking_periodval - t_rd_restval));
    | end
  function Trefval = getTref(synoutval, randNumsval, trelval, tabsval):
    | function Trefval = getTref(synoutval, randNumsval, trelval, tabsval)
    |     trel_k = min(trelval*100/synoutval,trelval);
    |     Trefval = single(tabsval - trel_k*log(randNumsval)); 
    | end
